simulink model "iliad_test"  (R2018b)
settings: Solver=FixedStepAuto  StartTime=0.0  StopTime=inf  FixedStep=0.01  RelTol=1e-3
values from neighbouring files (symbols this model uses):
  max_output_len = 4000    [iliad_init.m]    (also in iliad_test_init.m)
  pos_threshold = 0.01    [iliad_init.m]    (also in iliad_test_init.m = 0.1)
  q_left_init = [ 0.4352, -1.0289,  0.1226, -1.6992, -0.5845,  1.0377, -1.1276]'    [iliad_init.m]    (also in iliad_test_init.m = [0.1, 0.1, 0.1, 0, 0,  1, -1.5]')
  q_right_init = [-0.0000, -1.9509, -0.0000, -1.8703, -0.0000, -0.6711,  0.0000]'    [iliad_init.m]    (also in iliad_test_init.m = [0.1, 0.1, 0.1, 0, 0, -1,    0]')
  t_prova = [300,300;            300,300;            800,800;            800,800;            800,800]    [iliad_init.m]    (also in iliad_test_init.m)
libraries: robotlib x6, realtime_pacer_lib x2
settings Model: Creator=ed  LastModifiedBy=ed

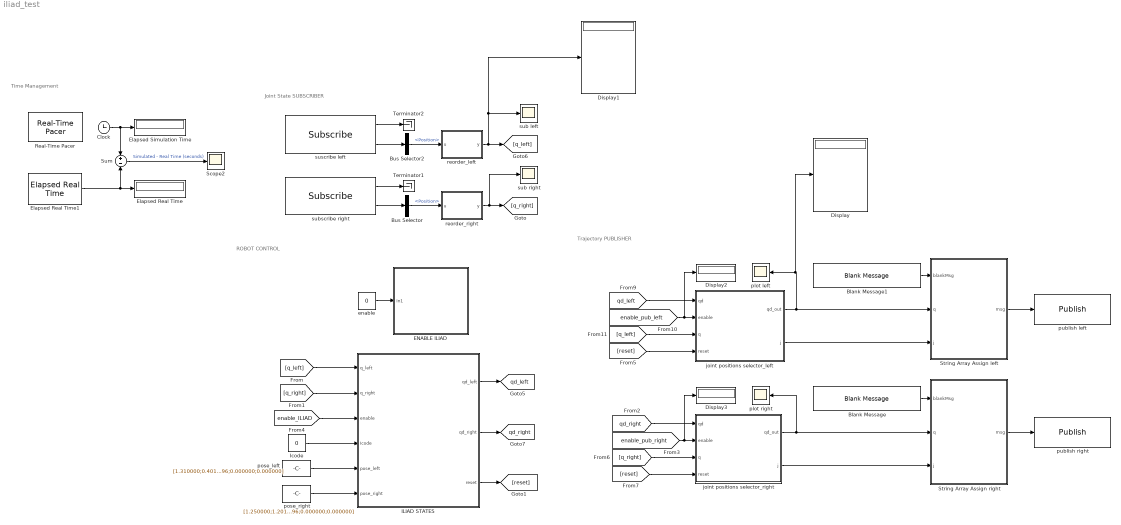
== system iliad_test ==
  note: ROBOT CONTROL
  note: Time Management
  note: Joint State SUBSCRIBER
  note: Trajectory PUBLISHER
  Blank Message : robotlib/Blank Message  messageClass=Message  entityType=sensor_msgs/JointState  messageType=sensor_msgs/JointState  SampleTime=-1
      settings: SourceProductBaseCode=RO
  Blank Message1 : robotlib/Blank Message  messageClass=Message  entityType=sensor_msgs/JointState  messageType=sensor_msgs/JointState  SampleTime=-1
      settings: SourceProductBaseCode=RO
  Bus Selector : BusSelector  OutputSignals=Position
  Bus Selector2 : BusSelector  OutputSignals=Position
  Clock : Clock
  Display{,1..3} (4 alike) : Display
  ENABLE ILIAD : Subsystem
  Elapsed Real Time : Display
      settings: Decimation=2
  Elapsed Real Time1 : realtime_pacer_lib/Elapsed Real Time
  Elapsed Simulation Time : Display
      settings: Decimation=2
  ILIAD STATES : Stateflow chart  TreatAsAtomicUnit=on
  Icode : Constant  Value=0
  Real-Time Pacer : realtime_pacer_lib/Real-Time Pacer  simTimePerRealTime=1
  Scope2 : Scope
  String Array Assign left : MATLAB Function  TreatAsAtomicUnit=on
  String Array Assign right : MATLAB Function  TreatAsAtomicUnit=on
  Sum : Sum  Inputs=+|-
  Terminator1 : Terminator
  Terminator2 : Terminator
  enable : Constant  Value=0
  joint positions selector_left : MATLAB Function  TreatAsAtomicUnit=on
  joint positions selector_right : MATLAB Function  TreatAsAtomicUnit=on
  plot left : Scope
  plot right : Scope
  pose_left : Constant  Value=[1.310000;0.401000;0.800000;-1.570796;0.000000;0.000000]
  pose_right : Constant  Value=[1.250000;1.201000;0.800000;-1.570796;0.000000;0.000000]
  publish left : robotlib/Publish  topicSource=Specify your own  topic=/left_arm/joint_states  messageType=sensor_msgs/JointState  messageQueueLength=1
      settings: SourceProductBaseCode=RO
  publish right : robotlib/Publish  topicSource=Specify your own  topic=/right_arm/joint_states  messageType=sensor_msgs/JointState  messageQueueLength=1
      settings: SourceProductBaseCode=RO
  reorder_left : MATLAB Function  TreatAsAtomicUnit=on
  reorder_right : MATLAB Function  TreatAsAtomicUnit=on
  sub left : Scope
  sub right : Scope
  subscribe right : robotlib/Subscribe  topicSource=Specify your own  topic=/right_arm/joint_states  messageType=sensor_msgs/JointState  sampleTime=-1  messageQueueLength=1
      settings: SourceProductBaseCode=RO
  suscribe left : robotlib/Subscribe  topicSource=Specify your own  topic=/left_arm/joint_states  messageType=sensor_msgs/JointState  sampleTime=-1  messageQueueLength=1
      settings: SourceProductBaseCode=RO
  tag scope: qd_left=global, qd_right=global
  wires:
  Sum/1 -> Scope2/1  "Simulated - Real Time (seconds)"
  Elapsed Real Time1/1 -> Sum/2, Elapsed Real Time/1
  Clock/1 -> Sum/1, Elapsed Simulation Time/1
  subscribe right/1 -> Terminator1/1
  suscribe left/2 -> Bus Selector2/1
  Bus Selector/1 -> reorder_right/1(u)  "<Position>"
  subscribe right/2 -> Bus Selector/1
  Blank Message/1 -> String Array Assign right/1(blankMsg)
  [q_right] -> joint positions selector_right/3(q)
  joint positions selector_left/1(qd_out) -> String Array Assign left/2(q), Display/1, plot left/1
  String Array Assign left/1(msg) -> publish left/1
  Blank Message1/1 -> String Array Assign left/1(blankMsg)
  joint positions selector_right/2(j) -> String Array Assign right/3(j)
  String Array Assign right/1(msg) -> publish right/1
  [q_left] -> joint positions selector_left/3(q)
  joint positions selector_right/1(qd_out) -> plot right/1, String Array Assign right/2(q)
  [qd_left] -> joint positions selector_left/1(qd)
  [qd_right] -> joint positions selector_right/1(qd)
  [enable_pub_right] -> joint positions selector_right/2(enable), Display3/1
  [enable_pub_left] -> joint positions selector_left/2(enable), Display2/1
  [q_left] -> ILIAD STATES/1(q_left)
  [q_right] -> ILIAD STATES/2(q_right)
  reorder_right/1(y) -> [q_right], sub right/1
  Bus Selector2/1 -> reorder_left/1(u)  "<Position>"
  reorder_left/1(y) -> [q_left], Display1/1, sub left/1
  suscribe left/1 -> Terminator2/1
  [enable_ILIAD] -> ILIAD STATES/3(enable)
  ILIAD STATES/2(qd_right) -> [qd_right]
  enable/1 -> ENABLE ILIAD/1(In1)
  ILIAD STATES/1(qd_left) -> [qd_left]
  joint positions selector_left/2(j) -> String Array Assign left/3(j)
  [reset] -> joint positions selector_right/4(reset)
  [reset] -> joint positions selector_left/4(reset)
  ILIAD STATES/3(reset) -> [reset]
  pose_left/1 -> ILIAD STATES/5(pose_left)
  pose_right/1 -> ILIAD STATES/6(pose_right)
  Icode/1 -> ILIAD STATES/4(Icode)

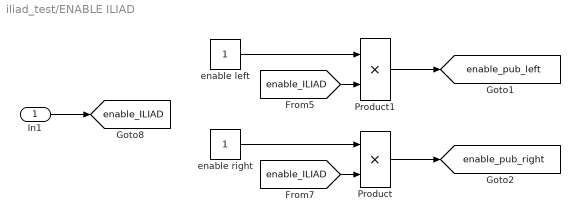
== system iliad_test/ENABLE ILIAD ==
  In1 : Inport
  Product : Product
  Product1 : Product
  enable left : Constant
  enable right : Constant
  tag scope: enable_ILIAD=global, enable_pub_left=global, enable_pub_right=global
  wires:
  enable left/1 -> Product1/1
  Product/1 -> [enable_pub_right]
  Product1/1 -> [enable_pub_left]
  In1/1 -> [enable_ILIAD]
  enable right/1 -> Product/1
  [enable_ILIAD] -> Product1/2
  [enable_ILIAD] -> Product/2

== matlab function iliad_test/joint positions selector_right ==
  data: qd input; enable input; qd_out output; j output; q input; reset input
function [qd_out, j] = publisher_(qd, enable, q, reset)
%% 
%qd_out = points to be send to the robot
%qd = entire trajectory generated by reverse priority
% enable = equal to 1 once a trajectpry qd has been generated by rev
% priority
%%
% if qd has been generated, this function selects consecutive joint
% positions along the trajectory qd to be send to the robot
persistent count 

if(isempty(count))
    count=1;
end

if reset
    count = 1;
end

qd_out = q;

if( enable == 1 )
   if (count > size(qd,2))
       count =  size(qd,2);
   end
   qd_out = qd(:,count);
   count = count + 1;
else
    qd_out = qd(:,count);
end
j = count;

end

== matlab function iliad_test/reorder_right ==
  data: u input; y output
function y = reorder(u)
%this function reorder joint position readings 
y = u(1:7);
% y(3) = u(7);
% for i = 4 : 7
%     y(i) = u(i-1);
% end

end

== matlab function iliad_test/reorder_left ==
  data: u input; y output
function y = reorder(u)
%this function reorder joint position readings 
y = u(1:7);
% y(3) = u(7);
% for i = 4 : 7
%     y(i) = u(i-1);
% end

end

== stateflow chart iliad_test/ILIAD STATES ==
  state homing
    en:
    coder.extrinsic('homing');
    coder.extrinsic('check_end_move')
    reset = 1;
    [qd_left, qd_right] = homing(q_curr_left, q_curr_right, t_prova, max_output_len);
    %% ----- %%
    du:
    reset = 0;
    flag_state = check_end_move(qd_left, qd_right, q_left, q_right, max_output_len, pos_threshold);
    %% ----- %%
    ex:
    q_curr_left = qd_left(:, end);
    q_curr_right = qd_right(:, end);
  state init
    en:
    qd_left   = repmat(q_left_init,   1, max_output_len );
    qd_right = repmat(q_right_init, 1, max_output_len );
    ex:
    q_curr_left = qd_left(:, end);
    q_curr_right = qd_right(:, end);
  state Go2Pose
    en:
    coder.extrinsic('go2pose');
    coder.extrinsic('check_end_move')
    reset = 1;
    [qd_left, qd_right] = go2pose(q_curr_left, q_curr_right, pose_right, pose_left, t_prova, max_output_len);
    %% ----- %%
    du:
    reset = 0;
    flag_state = check_end_move(qd_left, qd_right, q_left, q_right, max_output_len, pos_threshold);
    %% ----- %%
    ex:
    q_curr_left = qd_left(:, end);
    q_curr_right = qd_right(:, end);
  (default) -> init
  init -> homing : [enable == 1]{flag_state = 0}
  Go2Pose -> homing : [Icode == 0 && flag_state == 1]{flag_state = 0}
  homing -> Go2Pose : [Icode == 1 && flag_state == 1]{flag_state = 0}
  data: t_prova parameter; max_output_len parameter; q_left input size=[7 1]; q_right input size=[7 1]; enable input; Icode input; qd_left output size=[7 max_output_len]; qd_right output size=[7 max_output_len]; q_right_init parameter; q_curr_right local; q_curr_left local; pose_left input; reset output; pose_right input; flag_state local double size=1 =0; pos_threshold parameter; q_left_init parameter

== matlab function iliad_test/joint positions selector_left ==
  data: qd input; enable input; qd_out output; j output; q input; reset input
function [qd_out, j] = publisher_(qd, enable, q, reset)
%% 
%qd_out = points to be send to the robot
%qd = entire trajectory generated by reverse priority
% enable = equal to 1 once a trajectpry qd has been generated by rev
% priority
%%
% if qd has been generated, this function selects consecutive joint
% positions along the trajectory qd to be send to the robot
persistent count 

if(isempty(count))
    count = 1;
end

if reset
    count = 1;
end

qd_out = q;

if( enable == 1 )
   if (count > size(qd,2))
       count =  size(qd,2);
   end
   qd_out = qd(:,count);
   count = count + 1;
else
    qd_out = qd(:,count);
end
j = count;

end

== matlab function iliad_test/String Array Assign right ==
  data: blankMsg input; msg output Bus: SL_Bus_iliad_test_sensor_msgs_JointState; q input; j input
function msg = stringArrayAssign(blankMsg, q, j)
% stringArrayAssign - Assign a string array in a ROS message
%
%  blankMsg (input): A bus for a 'sensor_msgs/JointState' message. This is 
%                    used to initialize the output.
%  msg (output): A bus for a 'sensor_msgs/JointState' message message, with 
%                Name field set to a string array.
%
%  Copyleft 2015 The MathWorks, Inc.

% Note: The datatype of 'msg' has been explicitly set to the appropriate 
% Simulink bus type ("SL_Bus_robotROSMessageUsageExample_sensor_msgs_JointState"). 
%
% If the model name is changed, the datatype needs to be changed as well:
%   1) Click "Edit Data" in the Editor toolstrip to open "Ports and Data Manager"
%   2) Select "msg". From the "Type" dropdown, select "--- Refresh data types ---"
%   3) Set datatype to "Bus: SL_Bus_<modelname>_sensor_msgs_JointState"

strArrayToAssign = {'right_arm_a1_joint',...
                    'right_arm_a2_joint',...
                    'right_arm_e1_joint',...
                    'right_arm_a3_joint',...
                    'right_arm_a4_joint',...
                    'right_arm_a5_joint',...
                    'right_arm_a6_joint'};
msg = blankMsg;

numStringsInArray = length(strArrayToAssign);
msg.Name_SL_Info.CurrentLength = uint32(numStringsInArray);

% Set the individual strings in the array
for idx = 1 : numStringsInArray
    str = strArrayToAssign{idx};
    strLength = length(str);
    msg.Name(idx).Data(1:strLength) = uint8(str);
    msg.Name(idx).Data_SL_Info.CurrentLength = uint32(strLength);
end
msg.Position(1:length(q)) = q;
msg.Position_SL_Info.CurrentLength = uint32(length(q));

msg.Header.Seq = uint32(j);

== matlab function iliad_test/String Array Assign left ==
  data: blankMsg input; msg output Bus: SL_Bus_iliad_test_sensor_msgs_JointState; q input; j input
function msg = stringArrayAssign(blankMsg, q, j)
% stringArrayAssign - Assign a string array in a ROS message
%
%  blankMsg (input): A bus for a 'sensor_msgs/JointState' message. This is 
%                    used to initialize the output.
%  msg (output): A bus for a 'sensor_msgs/JointState' message message, with 
%                Name field set to a string array.
%
%  Copyleft 2015 The MathWorks, Inc.

% Note: The datatype of 'msg' has been explicitly set to the appropriate 
% Simulink bus type ("SL_Bus_robotROSMessageUsageExample_sensor_msgs_JointState"). 
%
% If the model name is changed, the datatype needs to be changed as well:
%   1) Click "Edit Data" in the Editor toolstrip to open "Ports and Data Manager"
%   2) Select "msg". From the "Type" dropdown, select "--- Refresh data types ---"
%   3) Set datatype to "Bus: SL_Bus_<modelname>_sensor_msgs_JointState"

strArrayToAssign = {'left_arm_a1_joint',...
                    'left_arm_a2_joint',...
                    'left_arm_e1_joint',... 
                    'left_arm_a3_joint',...
                    'left_arm_a4_joint',...
                    'left_arm_a5_joint',...
                    'left_arm_a6_joint'};
msg = blankMsg;

numStringsInArray = length(strArrayToAssign);
msg.Name_SL_Info.CurrentLength = uint32(numStringsInArray);

% Set the individual strings in the array
for idx = 1 : numStringsInArray
    str = strArrayToAssign{idx};
    strLength = length(str);
    msg.Name(idx).Data(1:strLength) = uint8(str);
    msg.Name(idx).Data_SL_Info.CurrentLength = uint32(strLength);
end
msg.Position(1:length(q)) = q;
msg.Position_SL_Info.CurrentLength = uint32(length(q));

msg.Header.Seq = uint32(j);
